simulink model "ex_2_2"  (R2024b)
settings: Solver=VariableStepAuto  StartTime=0.0  StopTime=10.0  RelTol=1e-3
values from neighbouring files (symbols this model uses):
  Nu = sol(n+1 : end)    [Script.m]
  Nx = sol(1 : n)    [Script.m]
  Ts = Ts_max / 4    (= 0.0218166156499)    [Script.m]
undefined symbols (not defined in the file or in its folder): A, A_obs, B, B_obs, C, C_obs, D, D_obs, k, step_amplitude
settings Model: Creator=andre  LastModifiedBy=farin

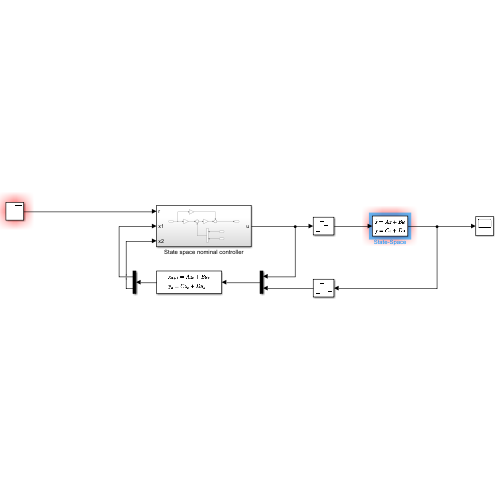
[thumbnail: Simulink's stored preview of the top-level diagram]
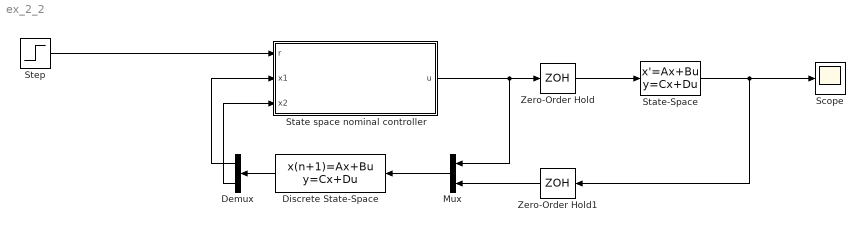
== system ex_2_2 ==
  Demux : Demux  Outputs=2
  Discrete State-Space : DiscreteStateSpace  A=A_obs  B=B_obs  C=C_obs  D=D_obs  SampleTime=Ts
  Mux : Mux  Inputs=2
  Scope : Scope
  State space nominal controller : Subsystem
  State-Space : StateSpace  A=A  B=B  C=C  D=D  InitialCondition=0
  Step : Step  Time=0  After=step_amplitude  SampleTime=0
  Zero-Order Hold : ZeroOrderHold  SampleTime=Ts
  Zero-Order Hold1 : ZeroOrderHold  SampleTime=Ts
  wires:
  State-Space/1 -> Zero-Order Hold1/1, Scope/1
  Zero-Order Hold/1 -> State-Space/1
  Zero-Order Hold1/1 -> Mux/2
  Mux/1 -> Discrete State-Space/1
  Discrete State-Space/1 -> Demux/1
  State space nominal controller/1(u) -> Mux/1, Zero-Order Hold/1
  Step/1 -> State space nominal controller/1(r)
  Demux/1 -> State space nominal controller/2(x1)
  Demux/2 -> State space nominal controller/3(x2)

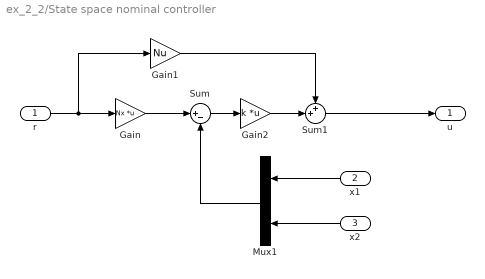
== system ex_2_2/State space nominal controller ==
  r : Inport
  x1 : Inport  Port=2
  x2 : Inport  Port=3
  Gain : Gain  Gain=Nx  Multiplication=Matrix(K*u)
  Gain1 : Gain  Gain=Nu
  Gain2 : Gain  Gain=k  Multiplication=Matrix(K*u)
  Mux1 : Mux  Inputs=2
  Sum : Sum  Inputs=|+-
  Sum1 : Sum  Inputs=++|
  u : Outport
  wires:
  Gain/1 -> Sum/1
  Sum1/1 -> u/1
  x1/1 -> Mux1/1
  r/1 -> Gain1/1, Gain/1
  Mux1/1 -> Sum/2
  Gain1/1 -> Sum1/1
  Sum/1 -> Gain2/1
  x2/1 -> Mux1/2
  Gain2/1 -> Sum1/2
